simulink model "sampleModel1597"  (R2023a)
settings: Solver=VariableStepAuto  StartTime=0.0  StopTime=10.0  RelTol=1e-3
libraries: hdlsllib x9, simulink x3
settings Model: Creator=user1  LastModifiedBy=user1

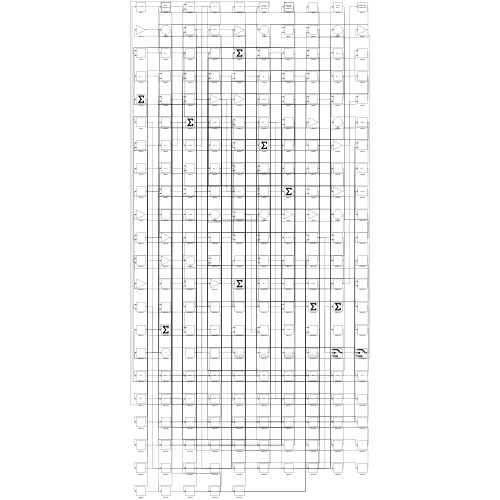
[thumbnail: Simulink's stored preview of the top-level diagram]
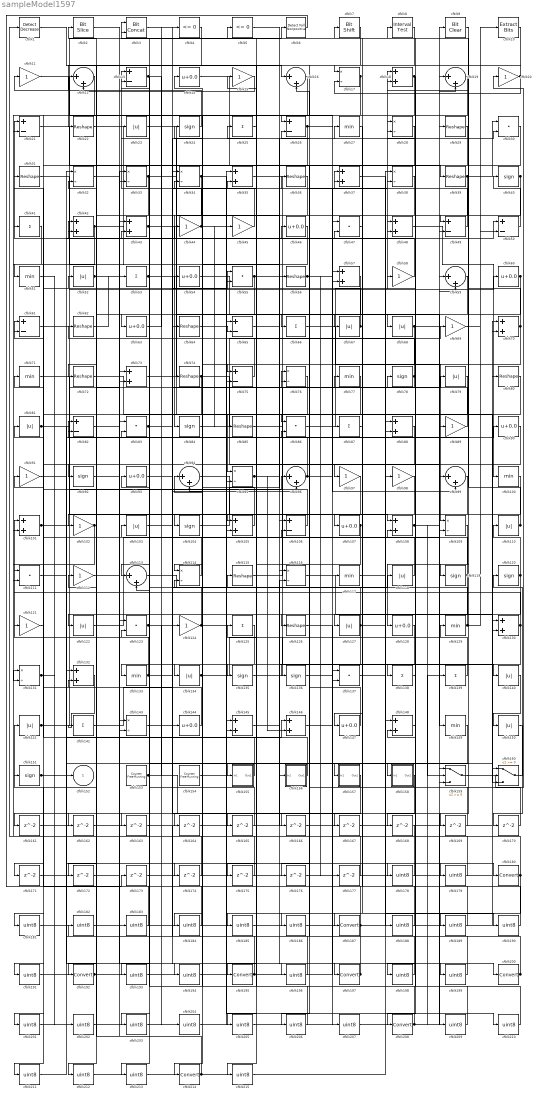
== system sampleModel1597 ==
  cfblk1 : simulink/Logic and Bit Operations/Detect Decrease  vinit=0.0  OutDataTypeStr=boolean
      settings: LibrarySourceBlock=|
      | hdlsllib/Logic and Bit
      | Operations/Detect
      | Decrease
  cfblk10 : simulink/Logic and Bit Operations/Extract Bits  bitsToExtract=Upper half  numBits=8  bitIdxRange=[0 7]  outScalingMode=Preserve fixed-point scaling
      settings: LibrarySourceBlock=|
      | hdlsllib/Logic and Bit
      | Operations/Extract Bits
  cfblk{27,51,71,77,100,117,129,133,149} (9 alike) : MinMax
  cfblk{18,35,37,42..43,48,57,70,73,88,101,105,108,130,132,145..146,148} (18 alike) : Sum
  cfblk{11,15,20,44..45,58,69,89,91,97..98,102,112,121,124} (15 alike) : Gain
  cfblk{23,52,67..68,79,81,103,110,118,122,127,134,140..141,150} (15 alike) : Abs  SaturateOnIntegerOverflow=off
  cfblk{24,40,78,84,92,104,119..120,135..136,151} (11 alike) : Signum
  cfblk{13,21,26,49..50,61,65,75,82,106} (10 alike) : Sum  Inputs=+-
  cfblk{14,46,54,60,63,90,93,107,128,144,147} (11 alike) : Bias  Bias=0.0  SaturateOnIntegerOverflow=off
  cfblk{17,28,32..34,38,76,95,109,114,116,131,143} (13 alike) : Product  Inputs=*/  RndMeth=Zero  SaturateOnIntegerOverflow=on
  cfblk{30,47,55,83,86,111,123,137} (8 alike) : DotProduct  OutDataTypeStr=Inherit: Inherit via internal rule
  cfblk{12,16,19,59,94,96,99,113} (8 alike) : Sum  Inputs=|++
  cfblk{22,29,31,36,39,56,62,64,72,74,80,85,115,126} (14 alike) : Reshape
  cfblk{25,41,53,66,87,125,138..139,142} (9 alike) : Sum  Inputs=+
  cfblk153 : hdlsllib/Sources/Counter Free-Running  NumBits=16  tsamp=-1
  cfblk154 : hdlsllib/Sources/Counter Free-Running  NumBits=16  tsamp=-1
  cfblk155 : Subsystem
      settings: LibrarySourceBlock=|
      | hdlsllib/Ports &
      | Subsystems/Subsystem
  cfblk156 : Subsystem
      settings: LibrarySourceBlock=|
      | hdlsllib/Ports &
      | Subsystems/Subsystem
  cfblk157 : Subsystem
      settings: LibrarySourceBlock=|
      | hdlsllib/Ports &
      | Subsystems/Subsystem
  cfblk158 : Subsystem
      settings: LibrarySourceBlock=|
      | hdlsllib/Ports &
      | Subsystems/Subsystem
  cfblk159 : Switch  SaturateOnIntegerOverflow=off  InputSameDT=off
  cfblk160 : Switch  SaturateOnIntegerOverflow=off  InputSameDT=off
  cfblk{161..177} (17 alike) : Delay  SampleTime=1
  cfblk{178..179,181..186,188..191,193..194,196,198..199,201..207,209..213,215} (30 alike) : DataTypeConversion  OutDataTypeStr=uint8  SaturateOnIntegerOverflow=off  RndMeth=Floor
  cfblk{180,187,192,195,197,200,208,214} (8 alike) : DataTypeConversion  SaturateOnIntegerOverflow=off  RndMeth=Floor
  cfblk2 : hdlsllib/Logic and Bit Operations/Bit Slice  lidx=7  ridx=0
  cfblk3 : hdlsllib/Logic and Bit Operations/Bit Concat  numInputs=2
  cfblk4 : hdlsllib/Logic and Bit Operations/Compare To Zero  relop=<=  OutDataTypeStr=boolean
  cfblk5 : hdlsllib/Logic and Bit Operations/Compare To Zero  relop=<=  OutDataTypeStr=boolean
  cfblk6 : hdlsllib/Logic and Bit Operations/Detect Fall Nonpositive  vinit=0  OutDataTypeStr=boolean
  cfblk7 : hdlsllib/Logic and Bit Operations/Bit Shift  mode=Shift Left Logical  N=0
  cfblk8 : hdlsllib/Logic and Bit Operations/Interval Test  IntervalClosedRight=on  uplimit=0.5  IntervalClosedLeft=on  lowlimit=-0.5  OutDataTypeStr=boolean
  cfblk9 : simulink/Logic and Bit Operations/Bit Clear  iBit=0
      settings: LibrarySourceBlock=|
      | hdlsllib/Logic and Bit
      | Operations/Bit Clear
  cfblk152 : Outport  VectorParamsAs1DForOutWhenUnconnected=off
  wires:
  cfblk41/1 -> cfblk51/1
  cfblk51/1 -> cfblk152/1
  cfblk69/1 -> cfblk10/1
  cfblk86/1 -> cfblk18/1
  cfblk90/1 -> cfblk141/1
  cfblk133/1 -> cfblk101/1, cfblk96/2, cfblk118/1
  cfblk27/1 -> cfblk97/1
  cfblk18/1 -> cfblk68/1, cfblk21/2
  cfblk63/1 -> cfblk4/1
  cfblk140/1 -> cfblk150/1
  cfblk60/1 -> cfblk164/1, cfblk165/1
  cfblk120/1 -> cfblk110/1, cfblk212/1
  cfblk55/1 -> cfblk138/1, cfblk105/2, cfblk15/1
  cfblk93/1 -> cfblk55/1
  cfblk115/1 -> cfblk77/1
  cfblk141/1 -> cfblk96/1, cfblk43/2
  cfblk12/1 -> cfblk101/2
  cfblk153/1 -> cfblk124/1, cfblk209/1
  cfblk34/1 -> cfblk84/1, cfblk210/1
  cfblk43/1 -> cfblk160/1, cfblk157/1(In1)
  cfblk9/1 -> cfblk119/1
  cfblk101/1 -> cfblk6/1, cfblk48/2
  cfblk66/1 -> cfblk109/1
  cfblk62/1 -> cfblk53/1
  cfblk52/1 -> cfblk102/1, cfblk179/1
  cfblk94/1 -> cfblk107/1
  cfblk50/1 -> cfblk40/1
  cfblk160/1 -> cfblk120/1
  cfblk23/1 -> cfblk95/1
  cfblk71/1 -> cfblk108/1
  cfblk2/1 -> cfblk73/1
  cfblk137/1 -> cfblk180/1
  cfblk74/1 -> cfblk109/2, cfblk181/1
  cfblk79/1 -> cfblk127/1
  cfblk24/1 -> cfblk11/1
  cfblk96/1 -> cfblk48/1, cfblk42/2
  cfblk54/1 -> cfblk66/1
  cfblk30/1 -> cfblk126/1
  cfblk118/1 -> cfblk81/1
  cfblk129/1 -> cfblk103/1, cfblk50/2
  cfblk138/1 -> cfblk8/1
  cfblk17/1 -> cfblk104/1, cfblk191/1
  cfblk128/1 -> cfblk134/1
  cfblk25/1 -> cfblk195/1
  cfblk139/1 -> cfblk129/1
  cfblk122/1 -> cfblk59/1
  cfblk40/1 -> cfblk49/1, cfblk158/1(In1)
  cfblk31/1 -> cfblk55/2
  cfblk125/1 -> cfblk133/1
  cfblk21/1 -> cfblk39/1
  cfblk35/1 -> cfblk149/1
  cfblk73/1 -> cfblk27/1
  cfblk83/1 -> cfblk78/1, cfblk86/1
  cfblk105/1 -> cfblk52/1
  cfblk159/1 -> cfblk20/1
  cfblk104/1 -> cfblk56/1
  cfblk48/1 -> cfblk100/1
  cfblk98/1 -> cfblk214/1
  cfblk84/1 -> cfblk69/1
  cfblk142/1 -> cfblk64/1
  cfblk154/1 -> cfblk65/1
  cfblk119/1 -> cfblk28/1, cfblk163/1
  cfblk7/1 -> cfblk72/1
  cfblk111/1 -> cfblk155/1(In1)
  cfblk13/1 -> cfblk63/1, cfblk204/1
  cfblk132/1 -> cfblk142/1
  cfblk42/1 -> cfblk156/1(In1), cfblk111/2
  cfblk26/1 -> cfblk99/2, cfblk161/1
  cfblk70/1 -> cfblk18/2, cfblk175/1
  cfblk47/1 -> cfblk187/1
  cfblk57/1 -> cfblk192/1
  cfblk65/1 -> cfblk28/2
  cfblk8/1 -> cfblk105/1
  cfblk22/1 -> cfblk74/1
  cfblk95/1 -> cfblk160/2, cfblk146/2, cfblk140/1
  cfblk44/1 -> cfblk13/1, cfblk67/1, cfblk85/1
  cfblk87/1 -> cfblk147/1
  cfblk148/1 -> cfblk208/1
  cfblk97/1 -> cfblk122/1
  cfblk53/1 -> cfblk95/2, cfblk30/2
  cfblk4/1 -> cfblk22/1
  cfblk99/1 -> cfblk114/1
  cfblk134/1 -> cfblk49/2, cfblk114/2
  cfblk102/1 -> cfblk131/2, cfblk172/1
  cfblk61/1 -> cfblk60/1
  cfblk109/1 -> cfblk128/1
  cfblk116/1 -> cfblk130/2
  cfblk106/1 -> cfblk71/1
  cfblk156/1(Out1) -> cfblk121/1
  cfblk20/1 -> cfblk17/1, cfblk17/2
  cfblk147/1 -> cfblk46/1
  cfblk146/1 -> cfblk50/1
  cfblk68/1 -> cfblk59/2, cfblk94/2
  cfblk76/1 -> cfblk113/1
  cfblk39/1 -> cfblk30/1, cfblk75/2
  cfblk123/1 -> cfblk3/1, cfblk167/1
  cfblk14/1 -> cfblk106/1
  cfblk75/1 -> cfblk62/1
  cfblk58/1 -> cfblk21/1
  cfblk151/1 -> cfblk146/1, cfblk90/1
  cfblk1/1 -> cfblk16/1
  cfblk107/1 -> cfblk136/1, cfblk205/1
  cfblk11/1 -> cfblk87/1
  cfblk59/1 -> cfblk135/1
  cfblk32/1 -> cfblk197/1
  cfblk108/1 -> cfblk99/1, cfblk159/2
  cfblk144/1 -> cfblk61/1
  cfblk155/1(Out1) -> cfblk113/2
  cfblk103/1 -> cfblk79/1
  cfblk124/1 -> cfblk42/1, cfblk37/2, cfblk24/1
  cfblk85/1 -> cfblk89/1
  cfblk72/1 -> cfblk144/1
  cfblk92/1 -> cfblk33/2
  cfblk82/1 -> cfblk73/2
  cfblk89/1 -> cfblk12/1
  cfblk10/1 -> cfblk26/1
  cfblk36/1 -> cfblk75/1
  cfblk78/1 -> cfblk23/1, cfblk76/2
  cfblk56/1 -> cfblk38/2, cfblk177/1
  cfblk15/1 -> cfblk12/2
  cfblk143/1 -> cfblk36/1
  cfblk45/1 -> cfblk14/1
  cfblk110/1 -> cfblk3/2, cfblk82/1
  cfblk81/1 -> cfblk43/1, cfblk174/1
  cfblk126/1 -> cfblk160/3
  cfblk114/1 -> cfblk41/1
  cfblk33/1 -> cfblk116/1, cfblk143/2
  cfblk127/1 -> cfblk76/1, cfblk176/1, cfblk186/1, cfblk189/1
  cfblk67/1 -> cfblk37/1, cfblk31/1
  cfblk38/1 -> cfblk92/1
  cfblk135/1 -> cfblk9/1
  cfblk113/1 -> cfblk115/1
  cfblk131/1 -> cfblk91/1, cfblk202/1
  cfblk64/1 -> cfblk65/2
  cfblk130/1 -> cfblk111/1, cfblk198/1
  cfblk145/1 -> cfblk200/1
  cfblk49/1 -> cfblk26/2
  cfblk121/1 -> cfblk61/2
  cfblk161/1 -> cfblk130/1
  cfblk28/1 -> cfblk162/1
  cfblk162/1 -> cfblk116/2
  cfblk164/1 -> cfblk94/1
  cfblk165/1 -> cfblk13/2
  cfblk3/1 -> cfblk166/1
  cfblk166/1 -> cfblk38/1
  cfblk167/1 -> cfblk159/1
  cfblk158/1(Out1) -> cfblk168/1
  cfblk168/1 -> cfblk1/1
  cfblk100/1 -> cfblk169/1
  cfblk169/1 -> cfblk106/2
  cfblk150/1 -> cfblk170/1
  cfblk170/1 -> cfblk108/2
  cfblk157/1(Out1) -> cfblk171/1
  cfblk171/1 -> cfblk33/1
  cfblk6/1 -> cfblk173/1
  cfblk173/1 -> cfblk70/1
  cfblk174/1 -> cfblk131/1
  cfblk175/1 -> cfblk34/2
  cfblk176/1 -> cfblk159/3
  cfblk177/1 -> cfblk16/2
  cfblk5/1 -> cfblk178/1
  cfblk178/1 -> cfblk54/1
  cfblk179/1 -> cfblk5/1
  cfblk180/1 -> cfblk82/2, cfblk7/1, cfblk215/1
  cfblk181/1 -> cfblk137/1
  cfblk182/1 -> cfblk137/2
  cfblk112/1 -> cfblk183/1
  cfblk183/1 -> cfblk83/1
  cfblk46/1 -> cfblk184/1
  cfblk184/1 -> cfblk112/1
  cfblk80/1 -> cfblk185/1
  cfblk185/1 -> cfblk70/2
  cfblk186/1 -> cfblk80/1
  cfblk187/1 -> cfblk182/1, cfblk151/1
  cfblk37/1 -> cfblk188/1
  cfblk188/1 -> cfblk47/1
  cfblk189/1 -> cfblk47/2
  cfblk117/1 -> cfblk190/1
  cfblk190/1 -> cfblk83/2
  cfblk191/1 -> cfblk117/1
  cfblk192/1 -> cfblk132/2, cfblk45/1
  cfblk16/1 -> cfblk193/1
  cfblk193/1 -> cfblk57/1
  cfblk172/1 -> cfblk194/1
  cfblk194/1 -> cfblk57/2
  cfblk195/1 -> cfblk123/2, cfblk125/1
  cfblk91/1 -> cfblk196/1
  cfblk196/1 -> cfblk25/1
  cfblk197/1 -> cfblk86/2, cfblk34/1
  cfblk198/1 -> cfblk32/1
  cfblk163/1 -> cfblk199/1
  cfblk199/1 -> cfblk32/2
  cfblk200/1 -> cfblk143/1, cfblk58/1
  cfblk77/1 -> cfblk201/1
  cfblk201/1 -> cfblk145/1
  cfblk202/1 -> cfblk145/2
  cfblk19/1 -> cfblk203/1
  cfblk203/1 -> cfblk35/1
  cfblk204/1 -> cfblk19/1
  cfblk205/1 -> cfblk19/2
  cfblk29/1 -> cfblk206/1
  cfblk206/1 -> cfblk44/1
  cfblk136/1 -> cfblk207/1
  cfblk207/1 -> cfblk29/1
  cfblk208/1 -> cfblk93/1, cfblk35/2, cfblk139/1
  cfblk209/1 -> cfblk148/1
  cfblk210/1 -> cfblk148/2
  cfblk88/1 -> cfblk211/1
  cfblk211/1 -> cfblk132/1
  cfblk212/1 -> cfblk88/1
  cfblk149/1 -> cfblk213/1
  cfblk213/1 -> cfblk88/2
  cfblk214/1 -> cfblk123/1, cfblk2/1
  cfblk215/1 -> cfblk98/1

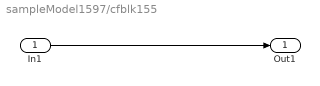
== system sampleModel1597/cfblk155 ==
  In1 : Inport
  Out1 : Outport
  wires:
  In1/1 -> Out1/1

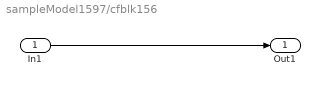
== system sampleModel1597/cfblk156 ==
  In1 : Inport
  Out1 : Outport
  wires:
  In1/1 -> Out1/1

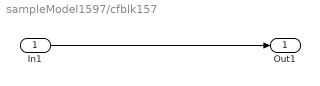
== system sampleModel1597/cfblk157 ==
  In1 : Inport
  Out1 : Outport
  wires:
  In1/1 -> Out1/1

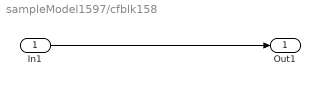
== system sampleModel1597/cfblk158 ==
  In1 : Inport
  Out1 : Outport
  wires:
  In1/1 -> Out1/1
